simulink model "Linear_Moving_Setpoint_SS_w_FF"  (R2021b)
settings: Solver=VariableStepAuto  StartTime=tspan(1)  StopTime=tspan(2)  RelTol=1e-7
undefined symbols (not defined in the file): K1, K2, r_sim
settings Model: Creator=domin  LastModifiedBy=domin
settings SolverCC: AlgebraicLoopSolver=TrustRegion
settings DebuggingCC: AlgebraicLoopMsg=none  SFMachineParentedDataDiag=warning

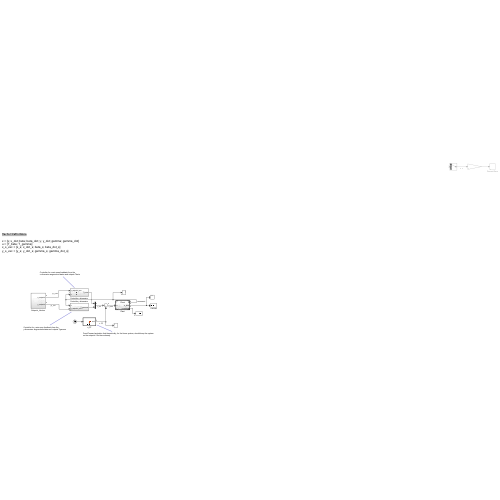
[thumbnail: Simulink's stored preview of the top-level diagram]
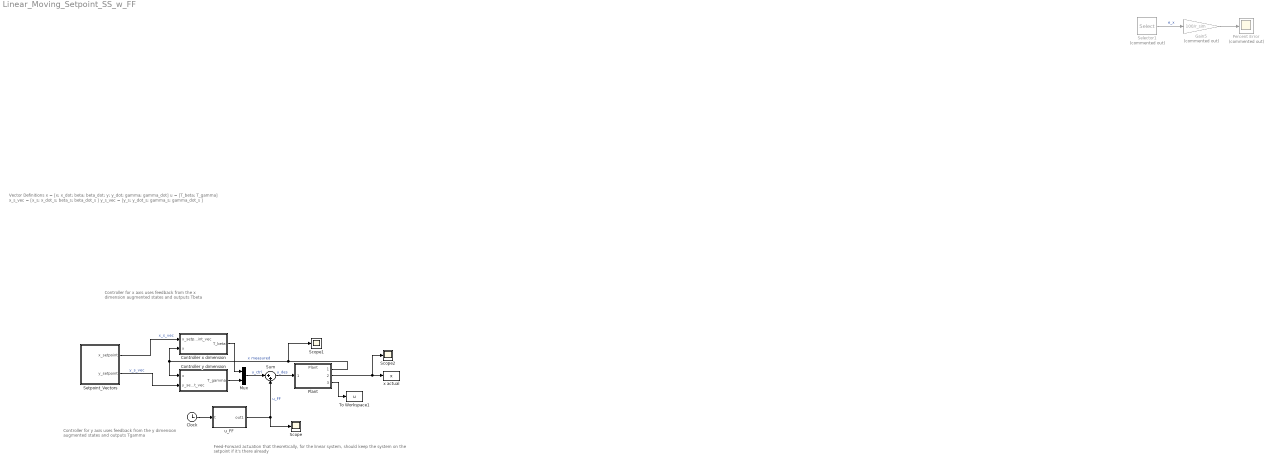
== system Linear_Moving_Setpoint_SS_w_FF ==
  note: Feed-Forward actuation that theoretically, for the linear system, should keep the system on the setpoint if it's there already
  note: Controller for y axis uses feedback from the
      | y dimension augmented states and outputs Tgamma
  note: Vector Definitions
      |
      | x = [x; x_dot; beta; beta_dot; y; y_dot; gamma; gamma_dot]
      | u = [T_beta; T_gamma]
      | x_s_vec = [x_s; x_dot_s; beta_s; beta_dot_s ]
      | y_s_vec = [y_s; y_dot_s; gamma_s; gamma_dot_s ]
  note: Controller for x axis uses feedback from the
      | x dimension augmented states and outputs Tbeta
  Clock : Clock
  Controller x dimension : Subsystem
  Controller y dimension : Subsystem
  Gain5 : Gain  Commented=on  Gain=100/r_sim
  Mux : Mux  Inputs=2
  Percent Error : Scope  Commented=on
  Plant : ModelReference  ModelNameDialog=Plant  SimulationMode=Normal  ModelReferenceVersion=1.104
  Scope : Scope
  Scope1 : Scope
  Scope2 : Scope
  Selector1 : Selector  Commented=on  InputPortWidth=5  IndexOptions=Index vector (dialog)  Indices=[1]  OutputSizes=1
  Setpoint_Vectors : Subsystem
  Sum : Sum  Inputs=|++
  To Workspace1 : ToWorkspace  VariableName=u  SampleTime=-1
  u_FF : MATLAB Function  TreatAsAtomicUnit=on
  x actual : ToWorkspace  VariableName=x  SampleTime=-1
  wires:
  Gain5/1 -> Percent Error/1
  Selector1/1 -> Gain5/1  "e_x"
  Controller x dimension/1(T_beta) -> Mux/1
  Controller y dimension/1(T_gamma) -> Mux/2
  Mux/1 -> Sum/1  "u_ctrl"
  Plant/1 -> Scope1/1, Controller x dimension/2(x), Controller y dimension/1(x)  "x measured"
  Plant/3 -> To Workspace1/1
  Plant/2 -> Scope2/1, x actual/1
  Setpoint_Vectors/1(x_setpoint) -> Controller x dimension/1(x_setpoint_vec)  "x_s_vec"
  Setpoint_Vectors/2(y_setpoint) -> Controller y dimension/2(y_setpoint_vec)  "y_s_vec"
  Clock/1 -> u_FF/1(t)
  Sum/1 -> Plant/1  "u_des"
  u_FF/1(out1) -> Scope/1, Sum/2  "u_FF"

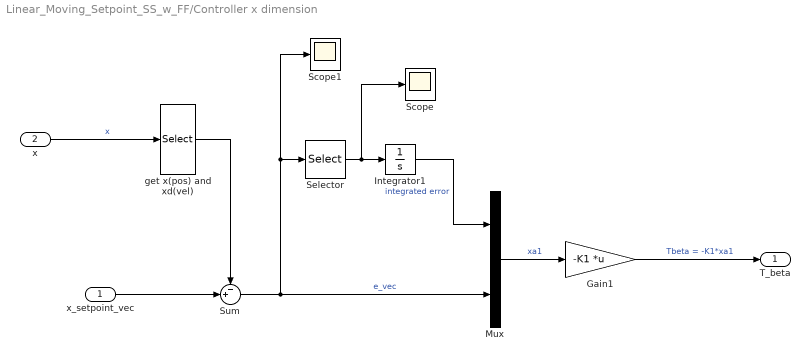
== system Linear_Moving_Setpoint_SS_w_FF/Controller x dimension ==
  x_setpoint_vec : Inport
  x : Inport  Port=2
  Gain1 : Gain  Gain=-K1  Multiplication=Matrix(K*u)
  Integrator1 : Integrator
  Mux : Mux  Inputs=2
  Scope : Scope
  Scope1 : Scope
  Selector : Selector  InputPortWidth=4  IndexOptions=Index vector (dialog)  Indices=[1 ]  OutputSizes=1
  Sum : Sum  Inputs=-+|
  get x(pos) and xd(vel) : Selector  InputPortWidth=8  IndexOptions=Index vector (dialog)  Indices=[1:4]  OutputSizes=1
  T_beta : Outport
  wires:
  Gain1/1 -> T_beta/1  "Tbeta = -K1*xa1"
  get x(pos) and xd(vel)/1 -> Sum/1
  Mux/1 -> Gain1/1  "xa1"
  Sum/1 -> Scope1/1, Selector/1, Mux/2  "e_vec"
  x_setpoint_vec/1 -> Sum/2
  x/1 -> get x(pos) and xd(vel)/1  "x"
  Selector/1 -> Scope/1, Integrator1/1
  Integrator1/1 -> Mux/1  "integrated error"

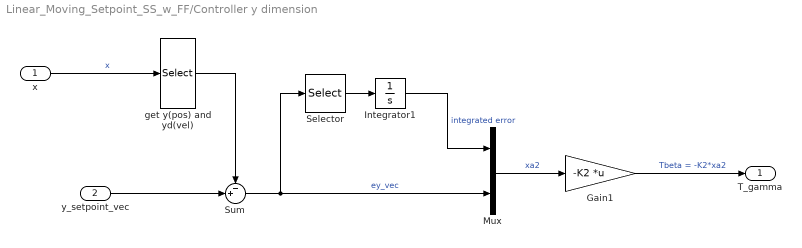
== system Linear_Moving_Setpoint_SS_w_FF/Controller y dimension ==
  x : Inport
  y_setpoint_vec : Inport  Port=2
  Gain1 : Gain  Gain=-K2  Multiplication=Matrix(K*u)
  Integrator1 : Integrator
  Mux : Mux  Inputs=2
  Selector : Selector  InputPortWidth=4  IndexOptions=Index vector (dialog)  Indices=[1 ]  OutputSizes=1
  Sum : Sum  Inputs=-+|
  get y(pos) and yd(vel) : Selector  InputPortWidth=8  IndexOptions=Index vector (dialog)  Indices=[5:8]  OutputSizes=1
  T_gamma : Outport
  wires:
  Integrator1/1 -> Mux/1  "integrated error"
  x/1 -> get y(pos) and yd(vel)/1  "x"
  Gain1/1 -> T_gamma/1  "Tbeta = -K2*xa2"
  get y(pos) and yd(vel)/1 -> Sum/1
  Mux/1 -> Gain1/1  "xa2"
  Selector/1 -> Integrator1/1
  Sum/1 -> Selector/1, Mux/2  "ey_vec"
  y_setpoint_vec/1 -> Sum/2

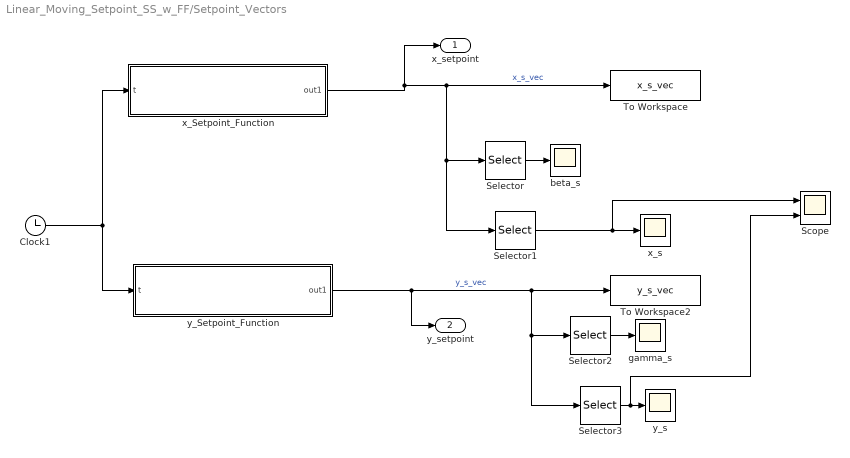
== system Linear_Moving_Setpoint_SS_w_FF/Setpoint_Vectors ==
  Clock1 : Clock
  Scope : Scope  NumInputPorts=2
  Selector : Selector  InputPortWidth=4  IndexOptions=Index vector (dialog)  Indices=[3]  OutputSizes=1
  Selector1 : Selector  InputPortWidth=4  IndexOptions=Index vector (dialog)  Indices=[1]  OutputSizes=1
  Selector2 : Selector  InputPortWidth=4  IndexOptions=Index vector (dialog)  Indices=[3]  OutputSizes=1
  Selector3 : Selector  InputPortWidth=4  IndexOptions=Index vector (dialog)  Indices=[1]  OutputSizes=1
  To Workspace : ToWorkspace  VariableName=x_s_vec  SampleTime=-1
  To Workspace2 : ToWorkspace  VariableName=y_s_vec  SampleTime=-1
  beta_s : Scope
  gamma_s : Scope
  x_Setpoint_Function : MATLAB Function  TreatAsAtomicUnit=on
  x_s : Scope
  y_Setpoint_Function : MATLAB Function  TreatAsAtomicUnit=on
  y_s : Scope
  x_setpoint : Outport
  y_setpoint : Outport  Port=2
  wires:
  Clock1/1 -> x_Setpoint_Function/1(t), y_Setpoint_Function/1(t)
  x_Setpoint_Function/1(out1) -> x_setpoint/1, Selector1/1, Selector/1, To Workspace/1  "x_s_vec"
  Selector/1 -> beta_s/1
  Selector1/1 -> Scope/1, x_s/1
  Selector3/1 -> Scope/2, y_s/1
  Selector2/1 -> gamma_s/1
  y_Setpoint_Function/1(out1) -> To Workspace2/1, Selector3/1, Selector2/1, y_setpoint/1  "y_s_vec"

== matlab function Linear_Moving_Setpoint_SS_w_FF/Setpoint_Vectors/x_Setpoint_Function ==
  data: t input; out1 output
function out1 = x_s_vec(t)
%#codegen

%    This function was generated by the Symbolic Math Toolbox version 9.0.
%    13-Mar-2022 23:59:22

t2 = pi.^2;
t3 = t.*2.0;
t6 = t.*pi.*(2.0./5.0);
t7 = t.*pi.*(6.0./5.0);
t4 = -t3;
t8 = cos(t6);
t9 = cos(t7);
t10 = sin(t6);
t11 = sin(t7);
t12 = t2.*1.298e+3;
t5 = exp(t4);
t14 = t12+6.8125e+4;
t13 = t5-1.0;
t15 = t14+5.45e+5;
t16 = 1.0./t14;
t17 = 1.0./t15;
t18 = t16.*5.510882126348228e+4;
t19 = t17.*4.959793913713405e+5;
t20 = t18-5.25e+2./6.49e+2;
t21 = t19-5.25e+2./6.49e+2;
out1 = [-t13.*(t8.*(3.0./4.0e+1)+t9.*(3.0./4.0e+1));t13.*(t10.*pi.*(3.0./1.0e+2)+t11.*pi.*(9.0./1.0e+2));-t13.*(t8.*t21+t9.*t20);t13.*(t10.*t21.*pi.*(2.0./5.0)+t11.*t20.*pi.*(6.0./5.0))];

== matlab function Linear_Moving_Setpoint_SS_w_FF/Setpoint_Vectors/y_Setpoint_Function ==
  data: t input; out1 output
function out1 = y_s_vec(t)
%#codegen

%    This function was generated by the Symbolic Math Toolbox version 9.0.
%    13-Mar-2022 23:59:22

t2 = pi.^2;
t3 = pi.^3;
t5 = pi.^5;
t6 = t.*2.0;
t9 = t.*pi.*(2.0./5.0);
t10 = t.*pi.*(6.0./5.0);
t16 = 3.76140931035164e+2;
t4 = t2.^2;
t7 = -t6;
t11 = cos(t9);
t12 = sin(t9);
t18 = t2.*8.842625e+8;
t19 = t.*t16.*(1.5e+1./6.49e+2);
t8 = exp(t7);
t14 = t12.^2;
t15 = t12.^3;
t17 = t4.*1.684804e+6;
t20 = -t19;
t21 = exp(t19);
t13 = t8-1.0;
t22 = exp(t20);
t23 = t17+t18+4.1769140625e+10;
t24 = t4.*t12.*t21.*2.7258e+6;
t25 = t4.*t15.*t21.*5.4516e+6;
t28 = t2.*t12.*t21.*1.8598125e+9;
t29 = t2.*t15.*t21.*2.575125e+9;
t26 = 1.0./t23;
t27 = -t25;
t30 = -t29;
t31 = t24+t27+t28+t30;
out1 = [t13.*(t12.*(3.0./4.0e+1)-sin(t10).*(3.0./4.0e+1));t13.*(t11.*pi.*(3.0./1.0e+2)-pi.*cos(t10).*(9.0./1.0e+2));-t13.*t22.*t26.*t31;-t13.*(t22.*t26.*(t3.*t11.*t21.*7.43925e+8+t5.*t11.*t21.*1.09032e+6-t3.*t11.*t14.*t21.*3.09015e+9+t2.*t12.*t16.*t21.*4.298488058551618e+7-t5.*t11.*t14.*t21.*6.54192e+6+t4.*t12.*t16.*t21.*6.3e+4-t2.*t15.*t16.*t21.*5.951752696456086e+7-t4.*t15.*t16.*t21.*1.26e+5)-t16.*t22.*t26.*t31.*(1.5e+1./6.49e+2))];

== matlab function Linear_Moving_Setpoint_SS_w_FF/u_FF ==
  data: out1 output size=2; t input
function out1 = u_FF(t)
%#codegen

%    This function was generated by the Symbolic Math Toolbox version 9.0.
%    13-Mar-2022 23:59:22

t2 = pi.^2;
t3 = pi.^3;
t5 = pi.^5;
t7 = t.*pi.*(2.0./5.0);
t8 = t.*pi.*(6.0./5.0);
t16 = 3.76140931035164e+2;
t4 = t2.^2;
t6 = t2.^3;
t9 = cos(t7);
t10 = cos(t8);
t11 = sin(t7);
t12 = t2.*1.298e+3;
t18 = t2.*8.842625e+8;
t22 = t.*t16.*(1.5e+1./6.49e+2);
t13 = t9.^2;
t14 = t11.^2;
t15 = t11.^3;
t17 = t4.*1.684804e+6;
t19 = t12+6.8125e+4;
t24 = -t22;
t25 = exp(t22);
t20 = t19+5.45e+5;
t21 = 1.0./t19;
t26 = exp(t24);
t29 = t17+t18+4.1769140625e+10;
t23 = 1.0./t20;
t27 = t21.*5.510882126348228e+4;
t30 = 1.0./t29;
t28 = t23.*4.959793913713405e+5;
t31 = t27-5.25e+2./6.49e+2;
t32 = t28-5.25e+2./6.49e+2;
et1 = t26.*t30.*(t2.*t11.*t25.*(-1.405605595146379e+11)+t4.*t11.*t25.*9.156e+7+t2.*t15.*t25.*1.94622313174114e+11+t6.*t11.*t25.*4.36128e+5-t4.*t15.*t25.*8.2404e+8-t6.*t15.*t25.*2.616768e+6-t3.*t9.*t16.*t25.*3.438790446841294e+7+t4.*t11.*t13.*t25.*2.47212e+9-t5.*t9.*t16.*t25.*5.04e+4+t6.*t11.*t13.*t25.*5.233536e+6+t3.*t9.*t14.*t16.*t25.*1.428420647149461e+8+t5.*t9.*t14.*t16.*t25.*3.024e+5);
et2 = -1.089342903606143e-1;
et3 = t11.*(-1.6554375e-1)+sin(t8).*1.6554375e-1+et1.*et2+t26.*t30.*(t2.*t11.*t25.*1.8598125e+9+t4.*t11.*t25.*2.7258e+6-t2.*t15.*t25.*2.575125e+9-t4.*t15.*t25.*5.4516e+6).*4.820308441084969;
et4 = t16.*t26.*t30.*(t3.*t9.*t25.*7.43925e+8+t5.*t9.*t25.*1.09032e+6-t3.*t9.*t14.*t25.*3.09015e+9-t5.*t9.*t14.*t25.*6.54192e+6+t2.*t11.*t16.*t25.*4.298488058551618e+7+t4.*t11.*t16.*t25.*6.3e+4-t2.*t15.*t16.*t25.*5.951752696456086e+7-t4.*t15.*t16.*t25.*1.26e+5).*(-5.035483375683249e-3);
out1 = [t9.*(-1.6554375e-1)-t10.*1.6554375e-1-t9.*t32.*3.412706878157143-t10.*t31.*3.412706878157143-t2.*t9.*t32.*1.742948645769829e-2-t2.*t10.*t31.*1.568653781192846e-1;et3+et4];
